simulink library "tsd"  (Simulink 8.1)
settings: Solver=ode1  StartTime=0.0  StopTime=Inf  FixedStep=0.001  RelTol=1e-3
PostLoadFcn:
  | , if any(exist('dsrtsu_mdlpostloadfcn', 'file') == [2, 3, 6]), try dsrtsu_mdlpostloadfcn('Execute', bdroot); catch fprintf('Error in PostLoadFcn (dsrtsu_mdlpostloadfcn) for model "%s":\n %s\n', bdroot, lasterr); end, end,
undefined symbols (not defined in the file or in its folder): C_TICK_TIME_S, FALSE, KIFO_TurnSignalTimer_ms, TRUE, ZERO_INT
libraries: hcu_lib x1
settings Model: DSRTSU_INTERNAL_RTI_VER=450  DSRTSU_INTERNAL_RTI_TYPE=rti1401  RTICANMMDATA=struct('GeneralSetupData',struct('modelroot','D:\ELN150201_TAIWAN\trunk\AdasDragon\software\sw_development\arch\app\ifo','generalsettings',struct('filesettings',struct('destfolder',struct('Name','RTICANMM_FILES','Check',1),'buildfolder',struct('Name','.','Check',1),'AbsDestfolder',struct('Name','D:\ELN150201_TAIWAN\trunk\AdasDragon\software\sw_development\arch\app\ifo\RTICANMM_FILES'),'AbsBuildfolder',struct('Name','D:\ELN150201_TAIWAN\trunk\AdasDragon\software\sw_development\arch\app\ifo'))),'options',struct('addpaths',1,'rmpaths',1,'addtrcexclusion',logical(1),'cannavigator',struct('checkmonitoring',0),'show_usrtrc',0,'use_usrtrc',0),'advanced',struct('options',[1 1 1 1 1 1 1 1 1 1 1 1 1 1 1 1 1 1 1 1 1 1 1 1 1 1 1 1 1 1 1 1 1 1 1 1 1 1 1 1 1 1 1 1 1 1 1 1 1 1 1 1 1 1 1 1 1 1 1 1 1 1 1 1 1 1 1 1 1 1 1 1 1 1 1 1 1 1 1 1 1 1 1 1 1 1 1 1 1 1 1 1 1 1 1 1 1 1 1 1]),'MPSetup',{{}},'modelname','tsd','block','tsd'))  DSRTSU_INTERNAL_RTIFPGA=40  Creator=AT015555  LastModifiedBy=AT015555

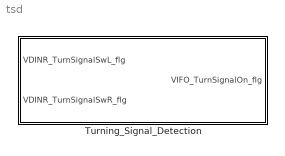
== system tsd ==
  Turning_Signal_Detection : Subsystem

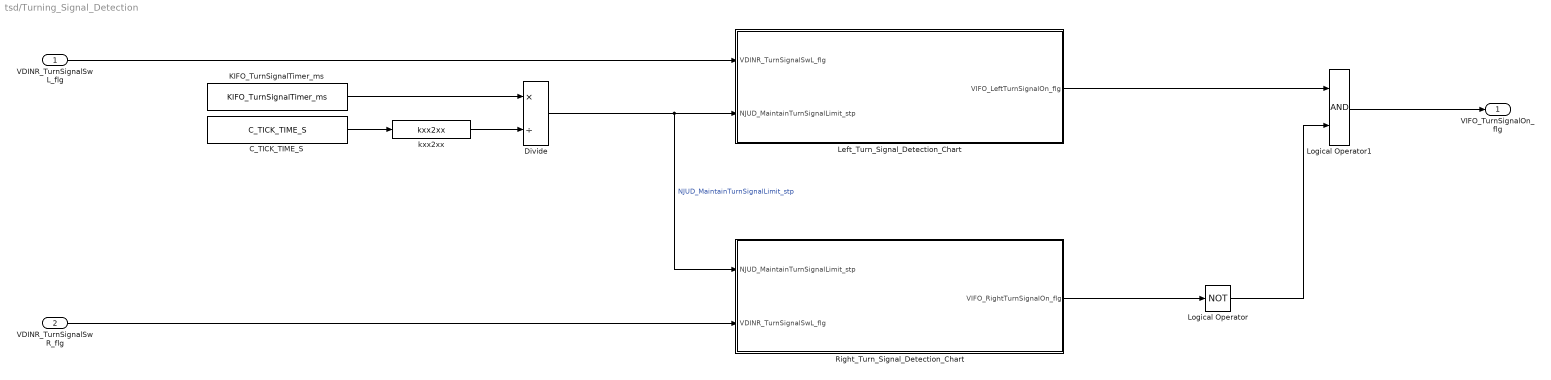
== system tsd/Turning_Signal_Detection ==
  VDINR_TurnSignalSwL_flg : Inport
  VDINR_TurnSignalSwR_flg : Inport  Port=2
  C_TICK_TIME_S : Constant  Value=C_TICK_TIME_S
  Divide : Product  Inputs=*/
  KIFO_TurnSignalTimer_ms : Constant  Value=KIFO_TurnSignalTimer_ms
  Left_Turn_Signal_Detection_Chart : Stateflow chart  TreatAsAtomicUnit=on
  Logical Operator : Logic  Operator=NOT  AllPortsSameDT=off  OutDataTypeStr=boolean
  Logical Operator1 : Logic  AllPortsSameDT=off  OutDataTypeStr=boolean
  Right_Turn_Signal_Detection_Chart : Stateflow chart  TreatAsAtomicUnit=on
  kxx2xx : hcu_lib/kxx2xx
  VIFO_TurnSignalOn_flg : Outport
  wires:
  Divide/1 -> Right_Turn_Signal_Detection_Chart/1(NJUD_MaintainTurnSignalLimit_stp), Left_Turn_Signal_Detection_Chart/2(NJUD_MaintainTurnSignalLimit_stp)  "NJUD_MaintainTurnSignalLimit_stp"
  KIFO_TurnSignalTimer_ms/1 -> Divide/1
  kxx2xx/1 -> Divide/2
  C_TICK_TIME_S/1 -> kxx2xx/1
  VDINR_TurnSignalSwL_flg/1 -> Left_Turn_Signal_Detection_Chart/1(VDINR_TurnSignalSwL_flg)
  Right_Turn_Signal_Detection_Chart/1(VIFO_RightTurnSignalOn_flg) -> Logical Operator/1
  Left_Turn_Signal_Detection_Chart/1(VIFO_LeftTurnSignalOn_flg) -> Logical Operator1/1
  Logical Operator/1 -> Logical Operator1/2
  Logical Operator1/1 -> VIFO_TurnSignalOn_flg/1
  VDINR_TurnSignalSwR_flg/1 -> Right_Turn_Signal_Detection_Chart/2(VDINR_TurnSignalSwL_flg)

== stateflow chart Turning_Signal_Detection/Left_Turn_Signal_Detection_Chart ==
  state OFF
    en:
    VIFO_LeftTurnSignalOn_flg = FALSE;
  state ON
    en:
    VIFO_LeftTurnSignalOn_flg = TRUE;
  state MAINTAIN
    en:
    NJUD_MaintainTurnSignalLocal_stp=ZERO_INT;
    du:
    NJUD_MaintainTurnSignalLocal_stp=NJUD_MaintainTurnSignalLocal_stp+1;
  (default) -> OFF
  OFF -> ON : [VDINR_TurnSignalSwL_flg==TRUE]
  (junction 14) -> OFF
  (junction 13) -> ON
  ON -> (junction 15)
  MAINTAIN -> (junction 13) [order 1] : [VDINR_TurnSignalSwL_flg==TRUE]
  MAINTAIN -> (junction 14) [order 2] : [NJUD_MaintainTurnSignalLocal_stp >= NJUD_MaintainTurnSignalLimit_stp]
  (junction 15) -> MAINTAIN : [VDINR_TurnSignalSwL_flg==FALSE]
  data: VDINR_TurnSignalSwL_flg input double; VIFO_LeftTurnSignalOn_flg output boolean; TRUE parameter boolean; FALSE parameter boolean; ZERO_INT parameter double; NJUD_MaintainTurnSignalLocal_stp local uint8; NJUD_MaintainTurnSignalLimit_stp input double

== stateflow chart Turning_Signal_Detection/Right_Turn_Signal_Detection_Chart ==
  state OFF
    en:
    VIFO_RightTurnSignalOn_flg = FALSE;
  state ON
    en:
    VIFO_RightTurnSignalOn_flg = TRUE;
  state MAINTAIN
    en:
    NJUD_MaintainTurnSignalLocal_stp=ZERO_INT;
    du:
    NJUD_MaintainTurnSignalLocal_stp=NJUD_MaintainTurnSignalLocal_stp+1;
  (default) -> OFF
  OFF -> ON : [VDINR_TurnSignalSwL_flg==TRUE]
  (junction 37) -> OFF
  (junction 36) -> ON
  ON -> (junction 38)
  MAINTAIN -> (junction 36) [order 1] : [VDINR_TurnSignalSwL_flg==TRUE]
  MAINTAIN -> (junction 37) [order 2] : [NJUD_MaintainTurnSignalLocal_stp >= NJUD_MaintainTurnSignalLimit_stp]
  (junction 38) -> MAINTAIN : [VDINR_TurnSignalSwL_flg==FALSE]
  data: NJUD_MaintainTurnSignalLimit_stp input double; VDINR_TurnSignalSwL_flg input double; VIFO_RightTurnSignalOn_flg output boolean; TRUE parameter boolean; FALSE parameter boolean; ZERO_INT parameter double; NJUD_MaintainTurnSignalLocal_stp local uint8
